simulink library "gps"  (R2016b)
settings: Solver=VariableStepAuto  StartTime=0.0  StopTime=10.0  RelTol=1e-3
undefined symbols (not defined in the file or in its folder): fsw_params
libraries: simulink x1
settings Model: Creator=bbarz_000  LastModifiedBy=taylorreynolds
settings OptimizationCC: LifeSpan=inf
settings DebuggingCC: SFExecutionAtInitializationDiag=none

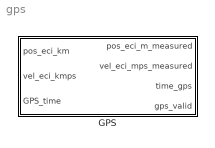
== system gps ==
  GPS : Subsystem

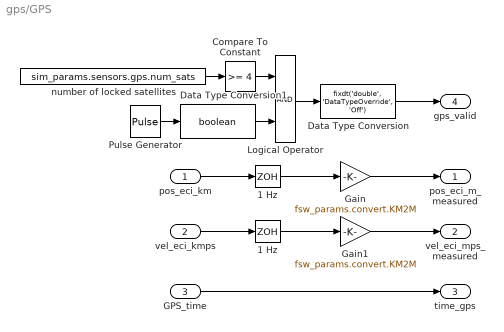
== system gps/GPS ==
  pos_eci_km : Inport
  vel_eci_kmps : Inport  Port=2
  GPS_time : Inport  Port=3
  1 Hz : ZeroOrderHold  SampleTime=0.2
  "1 Hz " : ZeroOrderHold  SampleTime=sim_params.sensors.gps.sample_time_s
  Compare To Constant : simulink/Logic and Bit Operations/Compare To Constant  relop=>=  const=4  OutDataTypeStr=boolean
  Data Type Conversion : DataTypeConversion  OutDataTypeStr=fixdt('double', 'DataTypeOverride', 'Off')  RndMeth=Nearest
  Data Type Conversion1 : DataTypeConversion  OutDataTypeStr=boolean  RndMeth=Nearest
  Gain : Gain  Gain=fsw_params.convert.KM2M
  Gain1 : Gain  Gain=fsw_params.convert.KM2M
  Logical Operator : Logic  AllPortsSameDT=off  OutDataTypeStr=boolean
  Pulse Generator : DiscretePulseGenerator  PulseType=Time based  Period=sim_params.sensors.gps.period  PulseWidth=sim_params.sensors.gps.pct_on  PhaseDelay=sim_params.sensors.gps.delay_s
  number of locked satellites : Constant  Value=sim_params.sensors.gps.num_sats
  pos_eci_m_measured : Outport
  vel_eci_mps_measured : Outport  Port=2
  time_gps : Outport  Port=3
  gps_valid : Outport  Port=4
  wires:
  Data Type Conversion1/1 -> Logical Operator/2
  Data Type Conversion/1 -> gps_valid/1
  Logical Operator/1 -> Data Type Conversion/1
  Pulse Generator/1 -> Data Type Conversion1/1
  pos_eci_km/1 -> 1 Hz/1
  vel_eci_kmps/1 -> "1 Hz "/1
  "1 Hz "/1 -> Gain1/1
  1 Hz/1 -> Gain/1
  number of locked satellites/1 -> Compare To Constant/1
  Compare To Constant/1 -> Logical Operator/1
  GPS_time/1 -> time_gps/1
  Gain/1 -> pos_eci_m_measured/1
  Gain1/1 -> vel_eci_mps_measured/1
